simulink model "CurrentSourceSimulation"  (Simulink 8.6)
settings: Solver=VariableStepAuto  StartTime=0.0  StopTime=0.5*10e-4  RelTol=1e-3
values from neighbouring files (symbols this model uses):
  c2_val = 200e-6    (= 0.0002)    [VoltageSourceController.m]    (also in main.m = 1e-06)
  C_ref = 10    [main.m]
  delay_load = t1    (= 3.6e-06)    [main.m]
  duty_inv = 100 - duty    (= 90)    [main.m]
  duty_load = (t2-t1)/T_mach*100    (= 8)    [main.m]
  f_sw = 500e3    (= 500000)    [main.m]
  fs2 = 2e3    (= 2000)    [VoltageSourceController.m]
  l1_val = 500e-4    (= 0.05)    [CurrentSourceController.m]    (also in main.m = 4.8e-07)
  l2_val = 50e-4    (= 0.005)    [VoltageSourceController.m]    (also in main.m = 1e-08)
  r_val = 1    [CurrentSourceController.m]    (also in VoltageSourceController.m; main.m)
  rc2_val = 0.0001    [main.m]
  rl1_val = 0.0002    [CurrentSourceController.m]    (also in main.m)
  rl2_val = 0.0001    [main.m]
  t2 = duty * T_mach / 100    (= 1.8e-05)    [main.m]
  T_mach = 180e-6    (= 0.00018)    [main.m]
  Vd_val = 100    [CurrentSourceController.m]    (also in VoltageSourceController.m = 8; main.m = 110)
libraries: powerlib x33, simulink x2, simulink_extras x2
settings Model: Creator=Akshay  LastModifiedBy=Akshay
settings SolverCC: ZeroCrossAlgorithm=Adaptive
settings DataIOCC: SaveFormat=Dataset  SignalLoggingSaveFormat=Dataset
settings OptimizationCC: ExpressionDepthLimit=128
settings DebuggingCC: UnderspecifiedInitializationDetection=Simplified  MergeDetectMultiDrivingBlocksExec=error  SolverPrmCheckMsg=none  FcnCallInpInsideContextMsg=EnableAllAsError  StateNameClashWarn=none
settings HardwareCC: ProdBitPerPointer=64  ProdLargestAtomicFloat=Float  ProdIntDivRoundTo=Zero  ProdEndianess=LittleEndian  ProdWordSize=64  ProdHWDeviceType=Intel->x86-64 (Windows64)
settings GRTTargetCC: GeneratePreprocessorConditionals=Use local settings  CombineOutputUpdateFcns=on  GRTInterface=off
settings ConfigComp: CovModelRefEnable=off

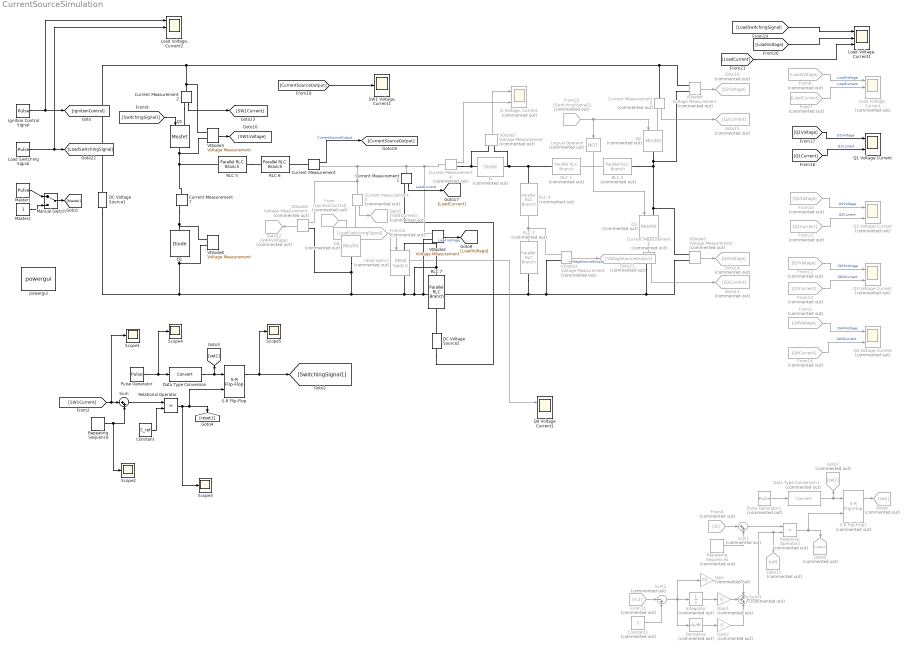
== system CurrentSourceSimulation ==
  " RLC 1" : powerlib/Elements/Parallel RLC Branch  Commented=on  LConnTagsString=a  RConnTagsString=__new0  BranchType=R  Resistance=rl2_val  Inductance=5e-6  SetiL0=off  InitialCurrent=0  Capacitance=0.3e-6  Setx0=off  InitialVoltage=0  Measurements=None
  " RLC 2" : powerlib/Elements/Parallel RLC Branch  Commented=on  LConnTagsString=a  RConnTagsString=__new0  BranchType=C  Resistance=1  Inductance=1e-3  SetiL0=off  InitialCurrent=0  Capacitance=c2_val  Setx0=off  InitialVoltage=50  Measurements=None
  " RLC 3" : powerlib/Elements/Parallel RLC Branch  Commented=on  LConnTagsString=a  RConnTagsString=__new0  BranchType=L  Resistance=50  Inductance=l2_val  SetiL0=off  InitialCurrent=0  Capacitance=0.3e-6  Setx0=off  InitialVoltage=0  Measurements=None
  " RLC 4" : powerlib/Elements/Parallel RLC Branch  Commented=on  LConnTagsString=a  RConnTagsString=__new0  BranchType=R  Resistance=rc2_val  Inductance=1e-3  SetiL0=off  InitialCurrent=0  Capacitance=0.1e-6  Setx0=off  InitialVoltage=0  Measurements=None
  " RLC 5" : powerlib/Elements/Parallel RLC Branch  LConnTagsString=a  RConnTagsString=__new0  BranchType=R  Resistance=rl1_val  Inductance=5e-6  SetiL0=off  InitialCurrent=0  Capacitance=0.3e-6  Setx0=off  InitialVoltage=0  Measurements=None
  " RLC 6" : powerlib/Elements/Parallel RLC Branch  LConnTagsString=a  RConnTagsString=__new0  BranchType=L  Resistance=50  Inductance=l1_val  SetiL0=off  InitialCurrent=100  Capacitance=0.3e-6  Setx0=off  InitialVoltage=0  Measurements=None
  " RLC 7" : powerlib/Elements/Parallel RLC Branch  LConnTagsString=a  RConnTagsString=__new0  BranchType=R  Resistance=r_val  Inductance=1e-3  SetiL0=off  InitialCurrent=0  Capacitance=0.1e-6  Setx0=off  InitialVoltage=0  Measurements=None
  Constant : Constant  Value=C_ref
  Constant1 : Constant  Commented=on  Value=5
  Current Measurement{,1..2,7} (4 alike) : powerlib/Measurements/Current Measurement  PhasorSimulation=off  OutputType=Complex  PSBequivalent=0
  Current Measurement{3..6} (4 alike) : powerlib/Measurements/Current Measurement  Commented=on  PhasorSimulation=off  OutputType=Complex  PSBequivalent=0
  D : powerlib/Power Electronics/Diode  Commented=on  Ron=0.001  Lon=0  Vf=0.8  IC=0  UseSnubber=off  Rs=500  Cs=250e-9  Measurements=off
  "D Voltage, Current" : Scope  Commented=on  NumInputPorts=2
  D1 : powerlib/Power Electronics/Diode  Ron=0.001  Lon=0  Vf=0.8  IC=0  UseSnubber=off  Rs=500  Cs=250e-9  Measurements=off
  DC Voltage Source1 : powerlib/Electrical Sources/DC Voltage Source  Amplitude=Vd_val  Measurements=Voltage
  DC Voltage Source2 : powerlib/Electrical Sources/DC Voltage Source  Amplitude=30  Measurements=Voltage
  Data Type Conversion : DataTypeConversion
  Data Type Conversion1 : DataTypeConversion  Commented=on
  Derivative : Derivative  Commented=on
  From : From  Commented=on  GotoTag=IgnitionControl
  From10 : From  Commented=on  GotoTag=Q2Voltage
  From11 : From  Commented=on  GotoTag=Q2Current
  From12 : From  Commented=on  GotoTag=Q3Voltage
  From13 : From  Commented=on  GotoTag=Q3Current
  From14 : From  Commented=on  GotoTag=QdCurrent
  From15 : From  Commented=on  GotoTag=vc2
  From22 : From  Commented=on  GotoTag=SwitchingSignal2
  From24 : From  Commented=on  GotoTag=LoadSwitchingSignal
  From3 : From  Commented=on  GotoTag=QdVoltage
  From4 : From  Commented=on  GotoTag=il2
  From6 : From  Commented=on  GotoTag=LoadVoltage
  From7 : From  Commented=on  GotoTag=LoadCurrent
  Gain : Gain  Commented=on  Gain=70
  Gain1 : Gain  Commented=on  Gain=0
  Gain2 : Gain  Commented=on  Gain=0
  Goto11 : Goto  Commented=on  GotoTag=ref
  Goto12 : Goto  Commented=on  GotoTag=SW4Voltage
  Goto13 : Goto  Commented=on  GotoTag=Q3Current
  Goto14 : Goto  Commented=on  GotoTag=Q3Voltage
  Goto15 : Goto  Commented=on  GotoTag=Q2Current
  Goto16 : Goto  Commented=on  GotoTag=Q2Voltage
  Goto21 : Goto  Commented=on  GotoTag=VoltageSourceOutput
  Goto5 : Goto  Commented=on  GotoTag=SW4Current
  Goto6 : Goto  Commented=on  GotoTag=sw2
  Goto7 : Goto  Commented=on  GotoTag=set2
  Goto8 : Goto  Commented=on  GotoTag=reset2
  Ideal Switch : powerlib/Power Electronics/Ideal Switch  Commented=on  Ron=0.001  Lon=0  IC=0  Rs=1e5  Cs=inf  Measurements=on
  Ignition Control Signal : DiscretePulseGenerator  PulseType=Time based  Period=T_mach  PulseWidth=duty_inv  PhaseDelay=t2
  Integrator : Integrator  Commented=on  ZeroCross=off
  Load Switching Signal : DiscretePulseGenerator  PulseType=Time based  Period=T_mach  PulseWidth=duty_load  PhaseDelay=delay_load
  "Load Voltage, Current" : Scope  Commented=on  NumInputPorts=3
  "Load Voltage, Current1" : Scope  NumInputPorts=3
  "Load Voltage, Current2" : Scope  NumInputPorts=3
  Logical Operator : Logic  Commented=on  Operator=NOT  AllPortsSameDT=off  OutDataTypeStr=boolean
  Manual Switch : ManualSwitch
  Master1 : DiscretePulseGenerator  PulseType=Time based  Period=180e-6  PulseWidth=6
  Master2 : Constant
  Pulse Generator : DiscretePulseGenerator  PulseType=Time based  Period=1/f_sw  PulseWidth=5
  Pulse Generator1 : DiscretePulseGenerator  Commented=on  PulseType=Time based  Period=1/fs2  PulseWidth=5
  Q1 : powerlib/Power Electronics/Mosfet  Ron=0.00001  Lon=0  Rd=0.0000000000001  Vfd=0  IC=0  Rs=1e5  Cs=inf  Measurements=off
  Q1 Voltage Current : Scope  NumInputPorts=2
  Q2 : powerlib/Power Electronics/Mosfet  Commented=on  Ron=0.00001  Lon=0  Rd=0.0000000000001  Vfd=0  IC=0  Rs=1e5  Cs=inf  Measurements=off
  Q2 Voltage Current : Scope  Commented=on  NumInputPorts=2
  Q3 : powerlib/Power Electronics/Mosfet  Commented=on  Ron=0.00001  Lon=0  Rd=0.0000000000001  Vfd=0  IC=0  Rs=1e5  Cs=inf  Measurements=off
  Q3 Voltage Current : Scope  Commented=on  NumInputPorts=2
  Qd : powerlib/Power Electronics/Mosfet  Commented=on  Ron=0.00001  Lon=0  Rd=0.0000000000001  Vfd=0  IC=0  Rs=1e5  Cs=inf  Measurements=off
  Qd Voltage Current : Scope  Commented=on  NumInputPorts=2
  Qd Voltage Current1 : Scope  NumInputPorts=2
  Relational Operator : RelationalOperator  Operator=>  OutDataTypeStr=boolean  ZeroCross=off
  Relational Operator1 : RelationalOperator  Commented=on  Operator=>  OutDataTypeStr=boolean  ZeroCross=off
  Repeating Sequence : simulink/Sources/Repeating Sequence  rep_seq_t=[0 1/f_sw]  rep_seq_y=[0 0]
  Repeating Sequence1 : simulink/Sources/Repeating Sequence  Commented=on  rep_seq_t=[0 1/fs2]  rep_seq_y=[0 0]
  S-R Flip-Flop : simulink_extras/Flip Flops/S-R Flip-Flop  initial_condition=0
  S-R Flip-Flop1 : simulink_extras/Flip Flops/S-R Flip-Flop  Commented=on  initial_condition=0
  "SW1 Voltage, Current1" : Scope
  Scope{1..5} (5 alike) : Scope
  Sum : Sum  Inputs=|++
  Sum1 : Sum  Commented=on  Inputs=|++
  Sum2 : Sum  Commented=on  Inputs=|-+
  Sum3 : Sum  Commented=on  Inputs=+++
  VDiode{1,4..7} (5 alike) : powerlib/Measurements/Voltage Measurement  Commented=on  PhasorSimulation=off  OutputType=Complex  PSBequivalent=0
  VDiode2 : powerlib/Measurements/Voltage Measurement  PhasorSimulation=off  OutputType=Complex  PSBequivalent=0
  VDiode3 : powerlib/Measurements/Voltage Measurement  PhasorSimulation=off  OutputType=Complex  PSBequivalent=0
  VDiode8 : powerlib/Measurements/Voltage Measurement  PhasorSimulation=off  OutputType=Complex  PSBequivalent=0
  powergui : powerlib/powergui  Priority=1  SimulationMode=Continuous  SolverType=Backward Euler  SampleTime=5e-07  frequency=60  SPID=on  DisableSnubberDevices=off  DisableRonSwitches=off  DisableVfSwitches=off  SwTol=0  DisplayEquations=off  Interpol=off  ExternalGateDelay=off  methode=off  Ts=0  FunctionMessages=off  echomessages=off  HookPort=off  EnableUseOfTLC=off  x0status=zero  frequencyindice=0  Pbase=100e6  ErrMax=1e-4  Iterations=50  UnitsV=kV  UnitsW=MW  buscounter=0  RestoreLinks=warning  ResistiveCurrentMeasurement=off  Frange=[0:2:500]  Ylog=off  Xlog=on  ShowGrid=off  save=off  variable=ZData  structure=ScopeData  ZoomFFT=off  StartTime=0.0  cycles=5  DisplayStyle=2  fundamental=50  FreqAxis=off  MaxFrequency=50000  frequencyindicesteady=1  RmsSteady=1  display=off
  wires:
  Pulse Generator/1 -> Scope4/1, Data Type Conversion/1
  Data Type Conversion/1 -> S-R Flip-Flop/1, [set1]
  Relational Operator/1 -> Scope3/1, S-R Flip-Flop/2, [reset1]
  S-R Flip-Flop/1 -> Scope5/1, [SwitchingSignal1]
  [SW1Current] -> Scope1/1, Sum/1
  Repeating Sequence/1 -> Scope2/1, Sum/2
  Sum/1 -> Relational Operator/1
  Constant/1 -> Relational Operator/2
  Pulse Generator1/1 -> Data Type Conversion1/1
  Data Type Conversion1/1 -> S-R Flip-Flop1/1, Goto7/1
  Relational Operator1/1 -> S-R Flip-Flop1/2, Goto8/1
  S-R Flip-Flop1/1 -> Goto6/1
  From4/1 -> Sum1/1
  Repeating Sequence1/1 -> Sum1/2
  Sum1/1 -> Relational Operator1/1
  From15/1 -> Sum2/1
  Constant1/1 -> Sum2/2
  Sum2/1 -> Derivative/1, Gain/1, Integrator/1
  Integrator/1 -> Gain1/1
  Gain1/1 -> Sum3/2
  Gain/1 -> Sum3/1
  Sum3/1 -> Relational Operator1/2, Goto11/1
  Derivative/1 -> Gain2/1
  Gain2/1 -> Sum3/3
  Logical Operator/1 -> Q3/1
  VDiode1/1 -> Goto21/1  "VoltageSourceOutput"
  Ignition Control Signal/1 -> [IgnitionControl], "Load Voltage, Current2"/1
  From/1 -> Qd/1
  VDiode2/1 -> [LoadVoltage]  "Load Voltage"
  Current Measurement1/1 -> [LoadCurrent]  "LoadCurrent"
  From6/1 -> "Load Voltage, Current"/1  "LoadVoltage"
  From7/1 -> "Load Voltage, Current"/2  "LoadCurrent"
  Current Measurement/1 -> [CurrentSourceOutput]  "CurrentSourceOutput"
  [SwitchingSignal1] -> Q1/1
  From22/1 -> Logical Operator/1, Q2/1
  Load Switching Signal/1 -> "Load Voltage, Current2"/2, [LoadSwitchingSignal]
  From24/1 -> Ideal Switch/1, Qd Voltage Current1/1
  Manual Switch/1 -> [Master]
  Master1/1 -> Manual Switch/1
  Master2/1 -> Manual Switch/2
  Current Measurement2/1 -> [SW1Current]
  VDiode3/1 -> [SW1Voltage]
  Current Measurement3/1 -> Goto5/1
  VDiode4/1 -> Goto12/1
  Current Measurement4/1 -> Goto13/1
  VDiode5/1 -> Goto14/1
  VDiode6/1 -> Goto16/1
  Current Measurement5/1 -> Goto15/1
  From10/1 -> Q2 Voltage Current/1  "Q2Voltage"
  From11/1 -> Q2 Voltage Current/2  "Q2Current"
  From12/1 -> Q3 Voltage Current/1  "SW3Voltage"
  From13/1 -> Q3 Voltage Current/2  "SW3Current"
  [Q1Voltage] -> Q1 Voltage Current/1  "Q1Voltage"
  [Q1Current] -> Q1 Voltage Current/2  "Q1Current"
  From3/1 -> Qd Voltage Current/1  "SW4Voltage"
  From14/1 -> Qd Voltage Current/2  "SW4Current"
  [CurrentSourceOutput] -> "SW1 Voltage, Current1"/1
  Current Measurement6/1 -> "D Voltage, Current"/2
  VDiode7/1 -> "D Voltage, Current"/1
  [LoadSwitchingSignal] -> "Load Voltage, Current1"/1
  [LoadVoltage] -> "Load Voltage, Current1"/2
  [LoadCurrent] -> "Load Voltage, Current1"/3
  connections:
  Q3/LConn1 -- VDiode5/LConn1 -- " RLC 3"/RConn1 -- Q2/RConn1 -- VDiode6/LConn2
  VDiode1/LConn1 -- " RLC 2"/LConn1 -- " RLC 4"/RConn1
  " RLC 1"/LConn1 -- " RLC 4"/LConn1 -- VDiode7/LConn2 -- D/RConn1
  Q1/RConn1 -- " RLC 5"/LConn1 -- Current Measurement7/LConn1 -- VDiode3/LConn2
  Current Measurement2/LConn1 -- VDiode3/LConn1 -- DC Voltage Source1/RConn1 -- Current Measurement5/LConn1 -- VDiode6/LConn1
  Current Measurement6/LConn1 -- VDiode2/LConn1 -- Current Measurement1/LConn1 -- VDiode4/LConn2 -- Current Measurement3/LConn1 -- Current Measurement/RConn1
  D/LConn1 -- Current Measurement6/RConn1 -- VDiode7/LConn1
  D1/RConn1 -- Current Measurement7/RConn1 -- VDiode8/LConn1
  " RLC 1"/RConn1 -- " RLC 3"/LConn1
  Current Measurement2/RConn1 -- Q1/LConn1
  Current Measurement3/RConn1 -- Qd/LConn1
  Current Measurement/LConn1 -- " RLC 6"/RConn1
  " RLC 5"/RConn1 -- " RLC 6"/LConn1
  DC Voltage Source2/RConn1 -- Current Measurement1/RConn1
  Current Measurement5/RConn1 -- Q2/LConn1
  VDiode2/LConn2 -- VDiode4/LConn1 -- Qd/RConn1 -- VDiode8/LConn2 -- D1/LConn1 -- DC Voltage Source1/LConn1 -- Ideal Switch/RConn1 -- Ideal Switch/LConn1 -- " RLC 7"/LConn1 -- Current Measurement4/RConn1 -- VDiode5/LConn2 -- VDiode1/LConn2 -- " RLC 2"/RConn1
  Current Measurement4/LConn1 -- Q3/RConn1
  DC Voltage Source2/LConn1 -- " RLC 7"/RConn1
